simulink subsystem "Lame"  (R2020a)
settings: Solver=VariableStepAuto  StartTime=0.0  StopTime=10.0  RelTol=1e-3
values from neighbouring files (symbols this model uses):
  g = 9.81    [default_design_data.mat]    (also in dict.sldd; modele_lame2.m)
  K_L = 0.004    [default_design_data.mat]    (also in dict.sldd)
  tau_L = 0.1    [default_design_data.mat]    (also in dict.sldd)
settings Model: Creator=frfoc1  LastModifiedBy=frfoc1

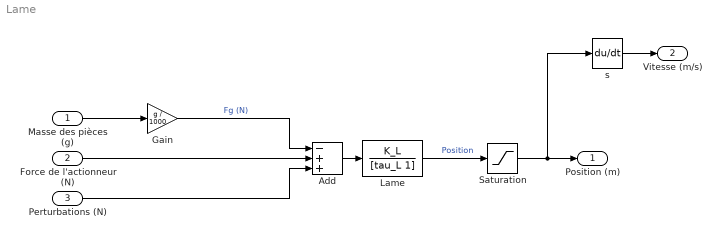
== system Lame ==
  Masse des pièces (g) : Inport
  "Force de l'actionneur (N) " : Inport  Port=2
  Perturbations (N) : Inport  Port=3
  Add : Sum  Inputs=-++
  Gain : Gain  Gain=g / 1000
  Lame : TransferFcn  Numerator=K_L  Denominator=[tau_L 1]
  Saturation : Saturate  UpperLimit=0.0031  LowerLimit=-0.0031
  s : Derivative
  Position (m) : Outport
  Vitesse (m/s) : Outport  Port=2
  wires:
  "Force de l'actionneur (N) "/1 -> Add/2
  Perturbations (N)/1 -> Add/3
  Gain/1 -> Add/1  "Fg (N)"
  Masse des pièces (g)/1 -> Gain/1
  Add/1 -> Lame/1
  Lame/1 -> Saturation/1  "Position"
  s/1 -> Vitesse (m/s)/1
  Saturation/1 -> Position (m)/1, s/1
